simulink model "bh_1dof_and_road_sim"  (R2021b)
settings: Solver=ode15s  StartTime=0.0  StopTime=30  MaxStep=0.001  RelTol=1e-5  EnableMultiTasking=on
undefined symbols (not defined in the file or in its folder): X, Y, Z
libraries: sm_lib x22, nesl_utility x6
Description:
  | Copyright 2014 The MathWorks, Inc.
settings Model: Creator=smiller  LastModifiedBy=bhorton
settings SolverCC: AlgebraicLoopSolver=TrustRegion
settings DataIOCC: LimitDataPoints=on  SaveFormat=Array  ReturnWorkspaceOutputs=off
settings OptimizationCC: LifeSpan=inf
settings DebuggingCC: UnderspecifiedInitializationDetection=Classic  MergeDetectMultiDrivingBlocksExec=none  SolverPrmCheckMsg=warning  AllowSymbolicDim=off  StateNameClashWarn=warning  SFUnexpectedBacktrackingDiag=warning  SFNoUnconditionalDefaultTransitionDiag=warning  SFExecutionAtInitializationDiag=none  SFMachineParentedDataDiag=warning  ArithmeticOperatorsInVariantConditions=warning
settings HardwareCC: ProdBitPerPointer=32  ProdBitPerSizeT=32  ProdBitPerPtrDiffT=32  ProdLargestAtomicFloat=None  ProdIntDivRoundTo=Undefined  ProdEndianess=Unspecified  ProdWordSize=32  ProdHWDeviceType=32-bit Generic
settings ModelReferenceCC: PropagateSignalLabelsOutOfModel=off
settings SFSimCC: SimUseLocalCustomCode=off  CustomCodeUndefinedFunction=UseInterfaceOnly
settings RTWCC: RTWUseLocalCustomCode=off
settings CodeAppCC: StateflowObjectComments=on
settings GRTTargetCC: TargetLangStandard=C89/C90 (ANSI)
settings ConfigComp: CovMetricSettings=dw  CovSaveCumulativeToWorkspaceVar=on  CovSaveSingleToWorkspaceVar=on  CovExternalEMLEnable=off  CovSFcnEnable=off
settings SimscapeCC: SimscapeNormalizeSystem=off
settings ExplorerConfigSet: InternalSimMechanicsExplorerSettings="<ExplorerConfiguration><canonicalview>default</canonicalview><AnimationSetting><BasePlaybackSpeed>1.0</BasePlaybackSpeed><PlaybackSpeedFactor>0.5</PlaybackSpeedFactor></AnimationSetting><TilePanel><TileInfo><Tiles Columns=\"1\" Count=\"1\" Rows=\"1\"><Column Weight=\"1\"/><Row Weight=\"1\"/><Tile Height=\"1\" Width=\"1\" X=\"0\" Y=\"0\"/></Tiles></TileInfo><SceneInfo><SceneViewer><BGColor><R>0.60000002384185791</R><G>0.60000002384185791</G><B>0.60000002384185791</B></BGColor><Camera><DoPerspective>on</DoPerspective><Position><X>0</X><Y>0</Y><Z>3</Z></Position><Center><X>0</X><Y>0</Y><Z>0</Z></Center><Up><X>0</X><Y>1</Y><Z>0</Z></Up><ViewLimDist>1</ViewLimDist><YLim>0.466307658154998583</YLim><XLim>0.517856281102247462</XLim></Camera></SceneViewer></SceneInfo></TilePanel><MechEditorPanel><Cameras><Camera><Id>Camera1</Id><Value><Name>Camera1</Name><NativeCamera><PositionTrackingFeature>THE_MODEL.CAR_ALTERNATE_MODEL_SIMSCAPE.RF_CAM.R</PositionTrackingFeature><CenterTrackingFeature>THE_MODEL.CAR_ALTERNATE_MODEL_SIMSCAPE.Road.R</CenterTrackingFeature><UpVectorTrackingFeature>THE_MODEL.CAR_ALTERNATE_MODEL_SIMSCAPE.RF1.R</UpVectorTrackingFeature><CenterTrackingOrigin>on</CenterTrackingOrigin><UpVectorTrackingDirection>+Y</UpVectorTrackingDirection></NativeCamera></Value></Camera></Cameras><GfxPanelCameraMap><MapElement CameraMLId=\"Camera1\" GfxPanelIndex=\"0\"/></GfxPanelCameraMap><VideoCreator><PlaybackSpeedRatio>4.0</PlaybackSpeedRatio><FrameRate>30</FrameRate><VideoFormat>MPEG-4</VideoFormat><FrameSize>[400 400]</FrameSize></VideoCreator></MechEditorPanel></ExplorerConfiguration>"

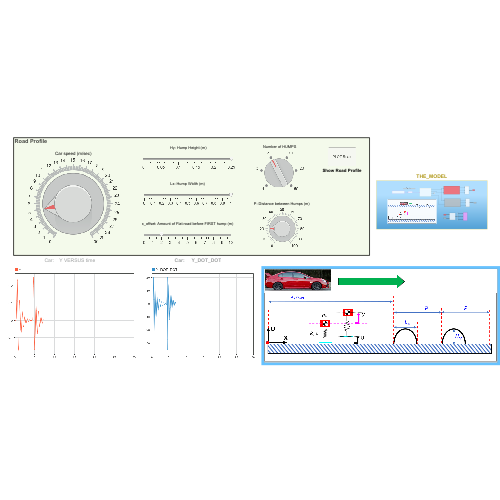
[thumbnail: Simulink's stored preview of the top-level diagram]
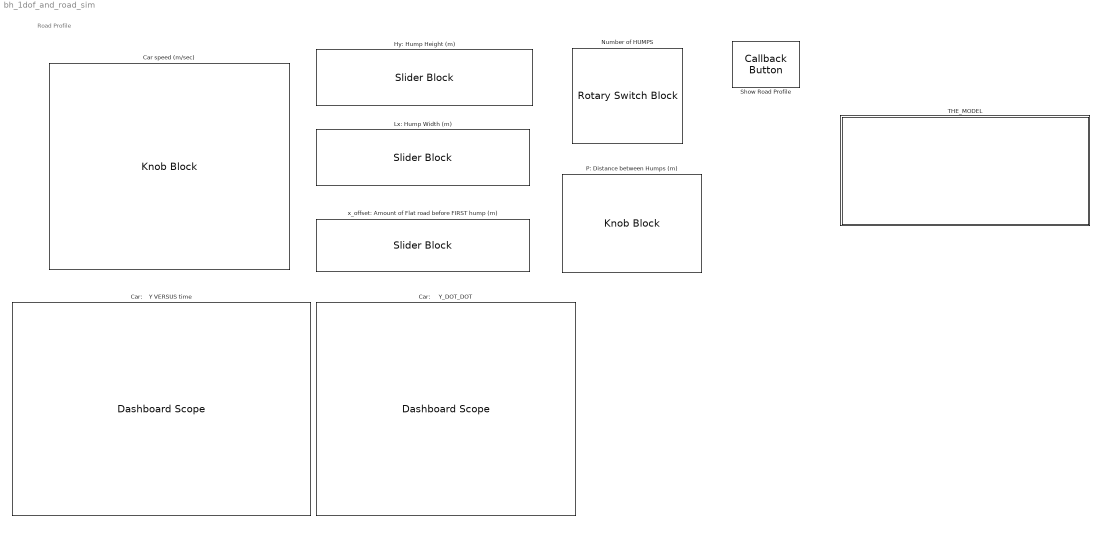
== system bh_1dof_and_road_sim ==
  note: Road Profile
  Car speed (m/sec) : KnobBlock  LabelPosition=Hide  ScaleMax=30  TickInterval=1
  Car:     Y_DOT_DOT : DashboardScope
  Car:    Y VERSUS time : DashboardScope
  Hy: Hump Height (m) : SliderBlock  LabelPosition=Hide  ScaleMax=0.25
  Lx: Hump Width (m) : SliderBlock  LabelPosition=Hide  ScaleMax=1
  Number of HUMPS : RotarySwitchBlock  LabelPosition=Hide
      settings: Values={{'1', '3', '5', '10', '20', '50'}, [1 3 5 10 20 50]}
  P: Distance between Humps (m) : KnobBlock  LabelPosition=Hide
  Show Road Profile : CallbackButton  ButtonText=PLOT Road
      settings: ClickFcn=bh_show_road_profile_from_Simulink(bdroot)
  THE_MODEL : Subsystem
  x_offset: Amount of Flat road before FIRST hump (m) : SliderBlock  LabelPosition=Hide  ScaleMax=10

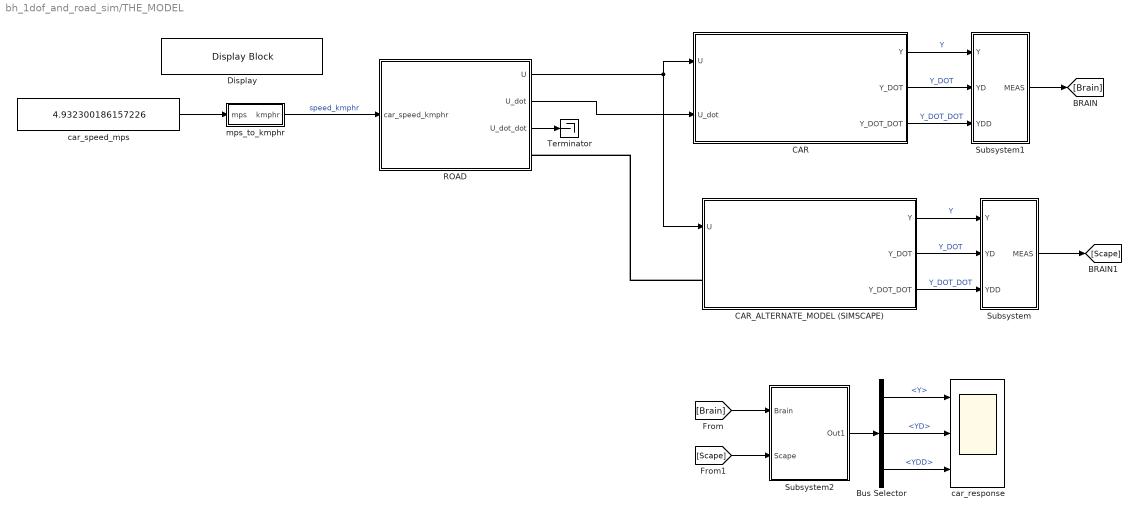
== system bh_1dof_and_road_sim/THE_MODEL ==
  Bus Selector : BusSelector  OutputSignals=Y,YD,YDD
  CAR : Subsystem  mask{m=5, c=2*10*0.6, k=500, y0=0, y_dot_0=0}
      mask prompts: m "m  (kg)"; c "c (N.s/m)"; k "k (N/m)"; y0 "y0 (m)"; y_dot_0 "y_dot_0  (m/s)"
      mask init:
      | str0 = sprintf('m  = %5.2f   (kg)', m);
      | str1 = sprintf('c  = %5.2f   (N.s/m)', c);
      | str2 = sprintf('k  = %5.2f   (N/m)', k);
      | str3 = sprintf('\n');
      | str4 = sprintf('y0 = %5.2f   (m)', y0);
      | str5 = sprintf('v0 = %5.2f   (m/s)', y_dot_0);
      | 
      | str  = char(str0,str1,str2,str3,str4,str5);
      mask DialogControl Container4 Prompt: M,C,K
      mask DialogControl Container3 Prompt: Initial Conditions
      mask Display: disp(str)
  CAR_ALTERNATE_MODEL (SIMSCAPE) : Subsystem  mask{m=5, c=2*10*0.6, k=500, y0=0, y_dot_0=0}
      mask prompts: m "m  (kg)"; c "c (N.s/m)"; k "k (N/m)"; y0 "y0 (m)"; y_dot_0 "y_dot_0  (m/s)"
      mask init: same as bh_1dof_and_road_sim/THE_MODEL/CAR
      mask DialogControl Container4 Prompt: M,C,K
      mask DialogControl Container3 Prompt: Initial Conditions
      mask Display: disp(str)
  Display : DisplayBlock  Format=short  Transparency=1
  ROAD : Subsystem  mask{m_Hy=0.25, m_Lx=1, m_P=20.15766016642253, m_x_offset=2, m_Np=5}
      mask prompts: m_Hy "Height of hump (m)"; m_Lx "Length of hump (m)"; m_P "Period of window (m)"; m_x_offset "X direction offset"; m_Np "Number of periods"
      mask init:
      | % create SYS object
      | OBJ = bh_road_hump_A_SYSO("Hy",m_Hy, "Lx",m_Lx, "P",m_P, ...
      |                           "x_offset",m_x_offset, "NUM_PERIODS",m_Np);
      |                       
      | tmp_x = linspace(0,(m_Np*m_P  +  m_x_offset), 1e4);
      | tmp_y = OBJ.get_y(tmp_x);
      | tmp_z = -2 * ones(size(tmp_x));
      | 
      | the_road_XYZ = [ tmp_x(:), tmp_y(:), tmp_z(:) ];
      mask DialogControl Control2 Prompt: Road Profile Parameters
  Subsystem : Subsystem
  Subsystem1 : Subsystem
  Subsystem2 : Subsystem
  Terminator : Terminator
  car_response : Scope  NumInputPorts=3
  car_speed_mps : Constant  Value=4.932300186157226
  mps_to_kmphr : Subsystem
  wires:
  ROAD/1(U) -> CAR/1(U), CAR_ALTERNATE_MODEL (SIMSCAPE)/1(U)
  car_speed_mps/1 -> mps_to_kmphr/1(mps)
  mps_to_kmphr/1(kmphr) -> ROAD/1(car_speed_kmphr)  "speed_kmphr"
  ROAD/2(U_dot) -> CAR/2(U_dot)
  ROAD/3(U_dot_dot) -> Terminator/1
  CAR_ALTERNATE_MODEL (SIMSCAPE)/1(Y) -> Subsystem/1(Y)  "Y"
  CAR_ALTERNATE_MODEL (SIMSCAPE)/2(Y_DOT) -> Subsystem/2(YD)  "Y_DOT"
  CAR_ALTERNATE_MODEL (SIMSCAPE)/3(Y_DOT_DOT) -> Subsystem/3(YDD)  "Y_DOT_DOT"
  CAR/1(Y) -> Subsystem1/1(Y)  "Y"
  CAR/2(Y_DOT) -> Subsystem1/2(YD)  "Y_DOT"
  CAR/3(Y_DOT_DOT) -> Subsystem1/3(YDD)  "Y_DOT_DOT"
  Subsystem1/1(MEAS) -> [Brain]
  Subsystem/1(MEAS) -> [Scape]
  [Brain] -> Subsystem2/1(Brain)
  [Scape] -> Subsystem2/2(Scape)
  Subsystem2/1(Out1) -> Bus Selector/1
  Bus Selector/1 -> car_response/1  "<Y>"
  Bus Selector/2 -> car_response/2  "<YD>"
  Bus Selector/3 -> car_response/3  "<YDD>"
  connections:
  CAR_ALTERNATE_MODEL (SIMSCAPE)/LConn1 -- ROAD/RConn1

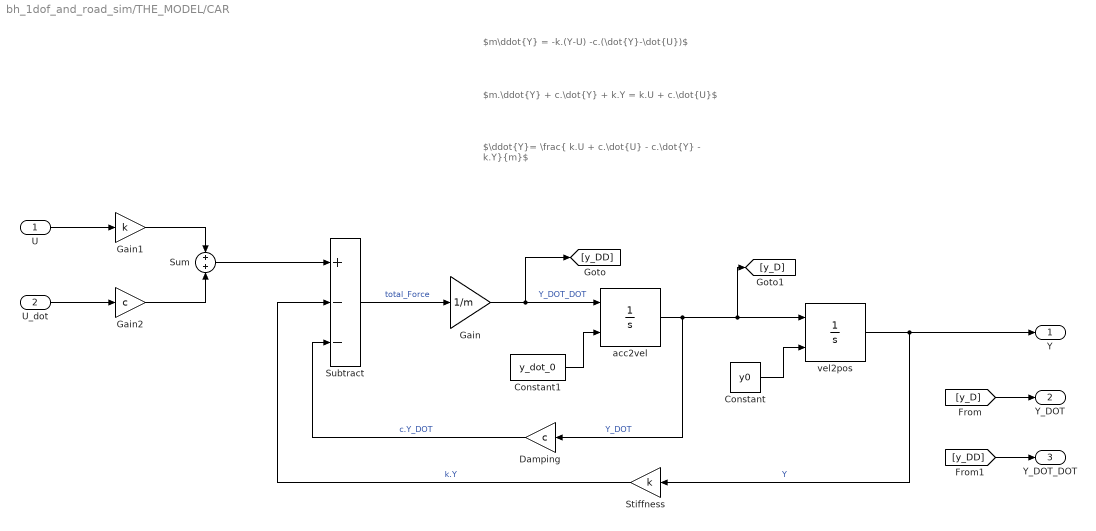
== system bh_1dof_and_road_sim/THE_MODEL/CAR ==
  note: $m.\ddot{Y} + c.\dot{Y} + k.Y = k.U + c.\dot{U}$
  note: $m\ddot{Y} = -k.(Y-U) -c.(\dot{Y}-\dot{U})$
  note: $\ddot{Y}= \frac{ k.U + c.\dot{U} - c.\dot{Y} - k.Y}{m}$
  U : Inport
  U_dot : Inport  Port=2
  Constant : Constant  Value=y0
  Constant1 : Constant  Value=y_dot_0
  Damping : Gain  Gain=c
  Gain : Gain  Gain=1/m
  Gain1 : Gain  Gain=k
  Gain2 : Gain  Gain=c
  Stiffness : Gain  Gain=k
  Subtract : Sum  Inputs=+--
  Sum : Sum  Inputs=+|+
  acc2vel : Integrator  InitialConditionSource=external
  vel2pos : Integrator  InitialConditionSource=external
  Y : Outport
  Y_DOT : Outport  Port=2
  Y_DOT_DOT : Outport  Port=3
  wires:
  Gain/1 -> [y_DD], acc2vel/1  "Y_DOT_DOT"
  Constant1/1 -> acc2vel/2
  Sum/1 -> Subtract/1
  Stiffness/1 -> Subtract/2  "k.Y"
  vel2pos/1 -> Y/1, Stiffness/1  "Y"
  Subtract/1 -> Gain/1  "total_Force"
  Constant/1 -> vel2pos/2
  acc2vel/1 -> [y_D], vel2pos/1, Damping/1  "Y_DOT"
  Damping/1 -> Subtract/3  "c.Y_DOT"
  U/1 -> Gain1/1
  U_dot/1 -> Gain2/1
  Gain1/1 -> Sum/1
  Gain2/1 -> Sum/2
  [y_D] -> Y_DOT/1
  [y_DD] -> Y_DOT_DOT/1

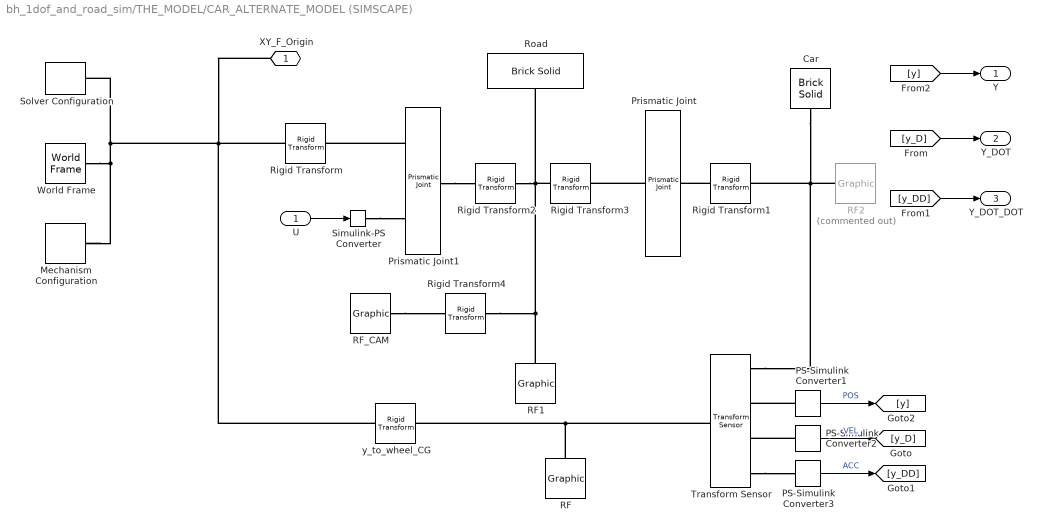
== system bh_1dof_and_road_sim/THE_MODEL/CAR_ALTERNATE_MODEL (SIMSCAPE) ==
  U : Inport
  Car : sm_lib/Body Elements/Brick Solid  GraphicAmbientColor=[0.15 0.15 0.15 1.0]  BasedOnType=Density  BrickDimensions=[1 1 1]*0.2  BrickDimensionUnits=m  CenterOfMass=[0 0 0]  CenterOfMassUnits=m  GraphicDiffuseColor=[1.0 0.2 0.2]  Density=1000  DensityUnits=kg/m^3  DoExposeReferenceFrame=on  GraphicEmissiveColor=[0.0 0.0 0.0 1.0]  ExportEntireGeometry=off  SerializedFrames=<Frames/>  MarkerShape=Sphere  MarkerSize=10  GraphicType=FromGeometry  InertiaType=PointMass  Mass=m  MassUnits=kg  MomentsOfInertia=[1 1 1]  MomentsOfInertiaUnits=kg*m^2  GraphicOpacity=1.0  ProductsOfInertia=[0 0 0]  ProductsOfInertiaUnits=kg*m^2  GraphicShininess=75  GraphicSpecularColor=[0.5 0.5 0.5 1.0]  GraphicVisPropType=SimpleVisualProperties
  Mechanism Configuration : sm_lib/Utilities/Mechanism Configuration  UniformGravity=Constant  GravityVector=[0 0 0]  GravityUnits=m/s^2  LinearizationDelta=0.001  JointModeTransitionNonlinearIterations=2
  PS-Simulink Converter1 : nesl_utility/PS-Simulink Converter  PhysicalDomain=network_engine_domain  SubClassName=ps_output  LeftPortType=input  RightPortType=output  PseudoPeriodic=off  Frequencies=[]  Unit=m  AffineConversion=off
      settings: SourceProductBaseCode=PW,SS
  PS-Simulink Converter2 : nesl_utility/PS-Simulink Converter  PhysicalDomain=network_engine_domain  SubClassName=ps_output  LeftPortType=input  RightPortType=output  PseudoPeriodic=off  Frequencies=[]  Unit=m/s  AffineConversion=off
      settings: SourceProductBaseCode=PW,SS
  PS-Simulink Converter3 : nesl_utility/PS-Simulink Converter  PhysicalDomain=network_engine_domain  SubClassName=ps_output  LeftPortType=input  RightPortType=output  PseudoPeriodic=off  Frequencies=[]  Unit=m/s^2  AffineConversion=off
      settings: SourceProductBaseCode=PW,SS
  Prismatic Joint : sm_lib/Joints/Prismatic Joint  JointMode=Normal  SenseConstraintForce=off  SenseConstraintForceX=off  SenseConstraintForceY=off  SenseConstraintForceZ=off  SenseConstraintTorque=off  SenseConstraintTorqueX=off  SenseConstraintTorqueY=off  SenseConstraintTorqueZ=off  SenseTotalForce=off  SenseTotalForceX=off  SenseTotalForceY=off  SenseTotalForceZ=off  SenseTotalTorque=off  SenseTotalTorqueX=off  SenseTotalTorqueY=off  SenseTotalTorqueZ=off  CompositeWrenchDir=FollowerOnBase  CompositeWrenchFrame=BaseFrame  EquilibriumPosition=1  EquilibriumPositionUnits=m  SpringStiffness=k  SpringStiffnessUnits=N/m  DampingCoefficient=c  DampingCoefficientUnits=N/(m/s)  TorqueActuationMode=NoTorque  MotionActuationMode=ComputedMotion  SensePosition=off  SenseVelocity=off  SenseAcceleration=off  SenseTorqueForce=off  SenseLowerLimitTorqueForce=off  SenseUpperLimitTorqueForce=off  LowerLimitSpecify=off  LowerLimitBound=-1  LowerLimitBoundUnits=m  LowerLimitStiffness=1e6  LowerLimitStiffnessUnits=N/m  LowerLimitDamping=1e3  LowerLimitDampingUnits=N/(m/s)  LowerLimitTransitionRegionWidth=1e-4  LowerLimitTransitionRegionWidthUnits=m  UpperLimitSpecify=off  UpperLimitBound=1  UpperLimitBoundUnits=m  UpperLimitStiffness=1e6  UpperLimitStiffnessUnits=N/m  UpperLimitDamping=1e3  UpperLimitDampingUnits=N/(m/s)  UpperLimitTransitionRegionWidth=1e-4  UpperLimitTransitionRegionWidthUnits=m  PositionTargetSpecify=on  PositionTargetPriority=High  PositionTargetValue=1 + y0  PositionTargetValueUnits=m  VelocityTargetSpecify=on  VelocityTargetPriority=High  VelocityTargetValue=y_dot_0  VelocityTargetValueUnits=m/s
      settings: AttributesFormatString=|
      | C = %<DampingCoefficient>
      | K = %<SpringStiffness>
      | L = %<EquilibriumPosition>
      | y0 =%<PositionTargetValue>
      | y_dot_0 = %<VelocityTargetValue>
  Prismatic Joint1 : sm_lib/Joints/Prismatic Joint  JointMode=Normal  SenseConstraintForce=off  SenseConstraintForceX=off  SenseConstraintForceY=off  SenseConstraintForceZ=off  SenseConstraintTorque=off  SenseConstraintTorqueX=off  SenseConstraintTorqueY=off  SenseConstraintTorqueZ=off  SenseTotalForce=off  SenseTotalForceX=off  SenseTotalForceY=off  SenseTotalForceZ=off  SenseTotalTorque=off  SenseTotalTorqueX=off  SenseTotalTorqueY=off  SenseTotalTorqueZ=off  CompositeWrenchDir=FollowerOnBase  CompositeWrenchFrame=BaseFrame  EquilibriumPosition=0  EquilibriumPositionUnits=m  SpringStiffness=0  SpringStiffnessUnits=N/m  DampingCoefficient=0  DampingCoefficientUnits=N/(m/s)  TorqueActuationMode=ComputedTorque  MotionActuationMode=InputMotion  SensePosition=off  SenseVelocity=off  SenseAcceleration=off  SenseTorqueForce=off  SenseLowerLimitTorqueForce=off  SenseUpperLimitTorqueForce=off  LowerLimitSpecify=off  LowerLimitBound=-1  LowerLimitBoundUnits=m  LowerLimitStiffness=1e6  LowerLimitStiffnessUnits=N/m  LowerLimitDamping=1e3  LowerLimitDampingUnits=N/(m/s)  LowerLimitTransitionRegionWidth=1e-4  LowerLimitTransitionRegionWidthUnits=m  UpperLimitSpecify=off  UpperLimitBound=1  UpperLimitBoundUnits=m  UpperLimitStiffness=1e6  UpperLimitStiffnessUnits=N/m  UpperLimitDamping=1e3  UpperLimitDampingUnits=N/(m/s)  UpperLimitTransitionRegionWidth=1e-4  UpperLimitTransitionRegionWidthUnits=m  PositionTargetSpecify=off  PositionTargetPriority=High  PositionTargetValue=0  PositionTargetValueUnits=m  VelocityTargetSpecify=off  VelocityTargetPriority=High  VelocityTargetValue=0  VelocityTargetValueUnits=m/s
  RF : sm_lib/Body Elements/Graphic  GraphicType=Marker  MarkerShape=Frame  MarkerSize=30  GraphicVisPropType=SimpleVisualProperties  GraphicDiffuseColor=[0.0 0.0 0.0]  GraphicSpecularColor=[0.5 0.5 0.5 1.0]  GraphicAmbientColor=[0.15 0.15 0.15 1.0]  GraphicEmissiveColor=[0.0 0.0 0.0 1.0]  GraphicShininess=75  GraphicOpacity=1.0
  RF1 : sm_lib/Body Elements/Graphic  GraphicType=Marker  MarkerShape=Frame  MarkerSize=30  GraphicVisPropType=SimpleVisualProperties  GraphicDiffuseColor=[0.0 0.0 0.0]  GraphicSpecularColor=[0.5 0.5 0.5 1.0]  GraphicAmbientColor=[0.15 0.15 0.15 1.0]  GraphicEmissiveColor=[0.0 0.0 0.0 1.0]  GraphicShininess=75  GraphicOpacity=1.0
  RF2 : sm_lib/Body Elements/Graphic  Commented=on  GraphicType=Marker  MarkerShape=Frame  MarkerSize=50  GraphicVisPropType=SimpleVisualProperties  GraphicDiffuseColor=[0.2 0.2 1.0]  GraphicSpecularColor=[0.5 0.5 0.5 1.0]  GraphicAmbientColor=[0.15 0.15 0.15 1.0]  GraphicEmissiveColor=[0.0 0.0 0.0 1.0]  GraphicShininess=75  GraphicOpacity=1.0
  RF_CAM : sm_lib/Body Elements/Graphic  GraphicType=Marker  MarkerShape=Frame  MarkerSize=30  GraphicVisPropType=SimpleVisualProperties  GraphicDiffuseColor=[0.0 0.0 0.0]  GraphicSpecularColor=[0.5 0.5 0.5 1.0]  GraphicAmbientColor=[0.15 0.15 0.15 1.0]  GraphicEmissiveColor=[0.0 0.0 0.0 1.0]  GraphicShininess=75  GraphicOpacity=1.0
  Rigid Transform : sm_lib/Frames and Transforms/Rigid Transform  TranslationMethod=None  TranslationStandardOffset=0  TranslationLengthUnit=m  TranslationStandardAxis=+Z  TranslationCartesianOffset=[0 0 0]  TranslationROffset=0  TranslationROffsetUnits=m  TranslationZOffset=0  TranslationZOffsetUnits=m  TranslationThetaOffset=0  TranslationThetaOffsetUnits=deg  RotationMethod=AlignedAxes  RotationAngleUnits=deg  RotationStandardAxis=+Z  RotationAngle=0.0  RotationArbitraryAxis=[0 0 1]  FollAlignAxisA=+Z  BaseAlignAxisA=+Y  FollAlignAxisB=+X  BaseAlignAxisB=+X  RotationSequenceAxes=FollowerAxes  RotationSequence=XYX  RotationSequenceAngles=[0 0 0]  RotationSequenceAnglesUnits=deg  RotationMatrix=[1 0 0; 0 1 0; 0 0 1]
  Rigid Transform1 : sm_lib/Frames and Transforms/Rigid Transform  TranslationMethod=None  TranslationStandardOffset=0  TranslationLengthUnit=m  TranslationStandardAxis=+Z  TranslationCartesianOffset=[0 0 0]  TranslationROffset=0  TranslationROffsetUnits=m  TranslationZOffset=0  TranslationZOffsetUnits=m  TranslationThetaOffset=0  TranslationThetaOffsetUnits=deg  RotationMethod=AlignedAxes  RotationAngleUnits=deg  RotationStandardAxis=+Z  RotationAngle=0.0  RotationArbitraryAxis=[0 0 1]  FollAlignAxisA=+Y  BaseAlignAxisA=+Z  FollAlignAxisB=+X  BaseAlignAxisB=+X  RotationSequenceAxes=FollowerAxes  RotationSequence=XYX  RotationSequenceAngles=[0 0 0]  RotationSequenceAnglesUnits=deg  RotationMatrix=[1 0 0; 0 1 0; 0 0 1]
  Rigid Transform2 : sm_lib/Frames and Transforms/Rigid Transform  TranslationMethod=None  TranslationStandardOffset=0  TranslationLengthUnit=m  TranslationStandardAxis=+Z  TranslationCartesianOffset=[0 0 0]  TranslationROffset=0  TranslationROffsetUnits=m  TranslationZOffset=0  TranslationZOffsetUnits=m  TranslationThetaOffset=0  TranslationThetaOffsetUnits=deg  RotationMethod=AlignedAxes  RotationAngleUnits=deg  RotationStandardAxis=+Z  RotationAngle=0.0  RotationArbitraryAxis=[0 0 1]  FollAlignAxisA=+Y  BaseAlignAxisA=+Z  FollAlignAxisB=+X  BaseAlignAxisB=+X  RotationSequenceAxes=FollowerAxes  RotationSequence=XYX  RotationSequenceAngles=[0 0 0]  RotationSequenceAnglesUnits=deg  RotationMatrix=[1 0 0; 0 1 0; 0 0 1]
  Rigid Transform3 : sm_lib/Frames and Transforms/Rigid Transform  TranslationMethod=None  TranslationStandardOffset=0  TranslationLengthUnit=m  TranslationStandardAxis=+Z  TranslationCartesianOffset=[0 0 0]  TranslationROffset=0  TranslationROffsetUnits=m  TranslationZOffset=0  TranslationZOffsetUnits=m  TranslationThetaOffset=0  TranslationThetaOffsetUnits=deg  RotationMethod=AlignedAxes  RotationAngleUnits=deg  RotationStandardAxis=+Z  RotationAngle=0.0  RotationArbitraryAxis=[0 0 1]  FollAlignAxisA=+Z  BaseAlignAxisA=+Y  FollAlignAxisB=+X  BaseAlignAxisB=+X  RotationSequenceAxes=FollowerAxes  RotationSequence=XYX  RotationSequenceAngles=[0 0 0]  RotationSequenceAnglesUnits=deg  RotationMatrix=[1 0 0; 0 1 0; 0 0 1]
  Rigid Transform4 : sm_lib/Frames and Transforms/Rigid Transform  TranslationMethod=StandardAxis  TranslationStandardOffset=3  TranslationLengthUnit=m  TranslationStandardAxis=+Z  TranslationCartesianOffset=[0 0 0]  TranslationROffset=0  TranslationROffsetUnits=m  TranslationZOffset=0  TranslationZOffsetUnits=m  TranslationThetaOffset=0  TranslationThetaOffsetUnits=deg  RotationMethod=None  RotationAngleUnits=deg  RotationStandardAxis=+Z  RotationAngle=0.0  RotationArbitraryAxis=[0 0 1]  FollAlignAxisA=+Y  BaseAlignAxisA=+Z  FollAlignAxisB=+X  BaseAlignAxisB=+X  RotationSequenceAxes=FollowerAxes  RotationSequence=XYX  RotationSequenceAngles=[0 0 0]  RotationSequenceAnglesUnits=deg  RotationMatrix=[1 0 0; 0 1 0; 0 0 1]
  Road : sm_lib/Body Elements/Brick Solid  GraphicAmbientColor=[0.15 0.15 0.15 1.0]  BasedOnType=Density  BrickDimensions=[0.2, 0.05, 0.2]  BrickDimensionUnits=m  CenterOfMass=[0 0 0]  CenterOfMassUnits=m  GraphicDiffuseColor=[0.0 1.0 1.0]  Density=1000  DensityUnits=kg/m^3  DoExposeReferenceFrame=on  GraphicEmissiveColor=[0.0 0.0 0.0 1.0]  ExportEntireGeometry=off  SerializedFrames=<Frames/>  MarkerShape=Sphere  MarkerSize=10  GraphicType=FromGeometry  InertiaType=PointMass  Mass=0.001  MassUnits=kg  MomentsOfInertia=[1 1 1]  MomentsOfInertiaUnits=kg*m^2  GraphicOpacity=1.0  ProductsOfInertia=[0 0 0]  ProductsOfInertiaUnits=kg*m^2  GraphicShininess=75  GraphicSpecularColor=[0.5 0.5 0.5 1.0]  GraphicVisPropType=SimpleVisualProperties
  Simulink-PS Converter : nesl_utility/Simulink-PS Converter  PhysicalDomain=network_engine_domain  SubClassName=ps_input  LeftPortType=input  RightPortType=output  PseudoPeriodic=off  Frequencies=[]  NoiseDistribution=none  NoiseParameters=[]  Unit=m  AffineConversion=off  FilteringAndDerivatives=filter  SimscapeFilterOrder=2  InputFilterTimeConstant=0.0005  UdotUserProvided=0
      settings: SourceProductBaseCode=PW,SS
  Solver Configuration : nesl_utility/Solver Configuration  PhysicalDomain=network_engine_domain  SubClassName=solver  LeftPortType=input  RightPortType=generic  Tones=[]  Harmonics=[]  SimulateNoise=off  Profile=off  UseLocalSampling=off  EnableSwitchedLinearOptims=on  FrequencyDomain=off  UseCCode=off  RelTol=0.001  AbsTol=1e-06  MinStep=1e-09  ToWorkspace=off  RevertToSquareIcSolve=off  NumHomotopyIterations=100  PhasorMode=off  PhasorModeNumHarmonics=1  DoDC=off  ResidualTolerance=1e-09  UseLocalSolver=off  LocalSolverChoice=NE_BACKWARD_EULER_ADVANCER  LocalSolverSampleTime=0.001  DoFixedCost=off  MaxNonlinIter=3  MaxModeIter=2  ComputeImpulses=off  ImpulseIterations=2  LinearAlgebra=Sparse  EquationFormulation=NE_TIME_EF  DelaysMemoryBudget=1024  AutomaticFiltering=on  FilteringTimeConstant=0.001  PartitionStorageMethod=AS_NEEDED  PartitionMemoryBudget=1024  PartitionMethod=FAST
      settings: SourceProductBaseCode=PW,SS
  Transform Sensor : sm_lib/Frames and Transforms/Transform Sensor  MeasurementFrame=World  SenseAngle=off  SenseAxis=off  SenseAngle1=off  SenseAngle2=off  SenseAngle3=off  SenseQ=off  SenseR=off  SenseOmegaX=off  SenseOmegaY=off  SenseOmegaZ=off  SenseOmega1=off  SenseOmega2=off  SenseOmega3=off  SenseQDot=off  SenseRDot=off  SenseAlphaX=off  SenseAlphaY=off  SenseAlphaZ=off  SenseAlpha1=off  SenseAlpha2=off  SenseAlpha3=off  SenseQDDot=off  SenseRDDot=off  SenseX=off  SenseY=on  SenseZ=off  SenseRad=off  SenseAzim=off  SenseDist=off  SenseInc=off  SenseXDot=off  SenseYDot=on  SenseZDot=off  SenseRadDot=off  SenseAzimDot=off  SenseDistDot=off  SenseIncDot=off  SenseXDDot=off  SenseYDDot=on  SenseZDDot=off  SenseRadDDot=off  SenseAzimDDot=off  SenseDistDDot=off  SenseIncDDot=off
  World Frame : sm_lib/Frames and Transforms/World Frame
  y_to_wheel_CG : sm_lib/Frames and Transforms/Rigid Transform  TranslationMethod=StandardAxis  TranslationStandardOffset=1  TranslationLengthUnit=m  TranslationStandardAxis=+Y  TranslationCartesianOffset="[-0.5,  1,  0]"  TranslationROffset=0  TranslationROffsetUnits=m  TranslationZOffset=0  TranslationZOffsetUnits=m  TranslationThetaOffset=0  TranslationThetaOffsetUnits=deg  RotationMethod=None  RotationAngleUnits=deg  RotationStandardAxis=+Z  RotationAngle=0.0  RotationArbitraryAxis=[0 0 1]  FollAlignAxisA=+Z  BaseAlignAxisA=+Y  FollAlignAxisB=+X  BaseAlignAxisB=+X  RotationSequenceAxes=FollowerAxes  RotationSequence=XYX  RotationSequenceAngles=[0 0 0]  RotationSequenceAnglesUnits=deg  RotationMatrix=[1 0 0; 0 1 0; 0 0 1]
      settings: AttributesFormatString=|
      | Axis = %<TranslationStandardAxis>
      | offset = %<TranslationStandardOffset>
  XY_F_Origin : PMIOPort  Side=Left
  Y : Outport
  Y_DOT : Outport  Port=2
  Y_DOT_DOT : Outport  Port=3
  wires:
  [y_D] -> Y_DOT/1
  [y_DD] -> Y_DOT_DOT/1
  PS-Simulink Converter2/1 -> [y_D]  "VEL"
  PS-Simulink Converter3/1 -> [y_DD]  "ACC"
  PS-Simulink Converter1/1 -> [y]  "POS"
  [y] -> Y/1
  U/1 -> Simulink-PS Converter/1
  connections:
  Prismatic Joint1/LConn1 -- Rigid Transform/RConn1
  Road/RConn1 -- Rigid Transform4/LConn1 -- RF1/RConn1 -- Rigid Transform2/RConn1 -- Rigid Transform3/LConn1
  Rigid Transform1/LConn1 -- Prismatic Joint/RConn1
  Car/RConn1 -- RF2/RConn1 -- Transform Sensor/RConn1 -- Rigid Transform1/RConn1
  y_to_wheel_CG/RConn1 -- Transform Sensor/LConn1 -- RF/RConn1
  PS-Simulink Converter1/LConn1 -- Transform Sensor/RConn2
  PS-Simulink Converter2/LConn1 -- Transform Sensor/RConn3
  Transform Sensor/RConn4 -- PS-Simulink Converter3/LConn1
  Simulink-PS Converter/RConn1 -- Prismatic Joint1/LConn2
  Prismatic Joint1/RConn1 -- Rigid Transform2/LConn1
  Prismatic Joint/LConn1 -- Rigid Transform3/RConn1
  Mechanism Configuration/RConn1 -- XY_F_Origin/RConn1 -- y_to_wheel_CG/LConn1 -- Rigid Transform/LConn1 -- Solver Configuration/RConn1 -- World Frame/RConn1
  RF_CAM/RConn1 -- Rigid Transform4/RConn1

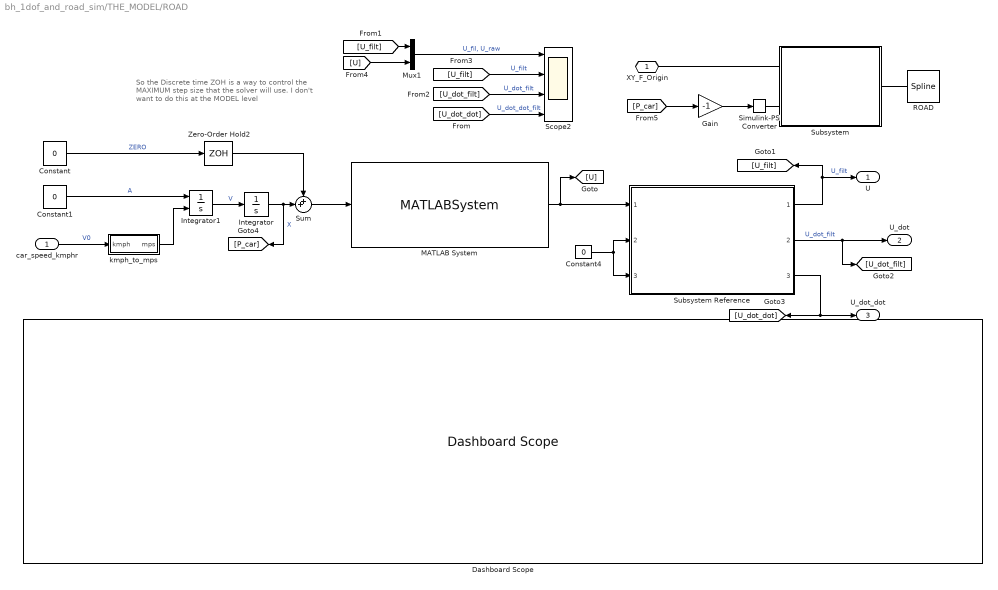
== system bh_1dof_and_road_sim/THE_MODEL/ROAD ==
  note: So the Discrete time ZOH is a way to control
      | the MAXIMUM step size that the solver will use.
      |
      | I don't want to do this at the MODEL level
  car_speed_kmphr : Inport
  Constant : Constant  Value=0
  Constant1 : Constant  Value=0
  Constant4 : Constant  Value=0
  Dashboard Scope : DashboardScope
  Gain : Gain  Gain=-1
  Integrator : Integrator
  Integrator1 : Integrator  InitialConditionSource=external
  MATLAB System : MATLABSystem  System=bh_road_hump_A_SYSO  Hy=m_Hy  Lx=m_Lx  P=m_P  x_offset=m_x_offset  NUM_PERIODS=m_Np  SimulateUsing=Interpreted execution
      mask Type: bh_road_hump_A_SYSO
      mask Display:
      | disp('bh_road_hump_A_SYSO');
      | port_label('input',1,'X_car');
      | port_label('output',1,'Y_road');
  Mux1 : Mux  Inputs=2
  ROAD : sm_lib/Curves and Surfaces/Spline  GraphicAmbientColor=[0.15 0.15 0.15 1.0]  GraphicDiffuseColor=[0.2 1.0 0.2]  DataPoints=the_road_XYZ  DataPointsUnits=m  GraphicEmissiveColor=[0.0 0.0 0.0 1.0]  EndConditionType=Natural  MarkerShape=Sphere  MarkerSize=10  GraphicType=FromGeometry  GraphicOpacity=1.0  GraphicShininess=75  GraphicSpecularColor=[0.5 0.5 0.5 1.0]  GraphicVisPropType=SimpleVisualProperties
  Scope2 : Scope  NumInputPorts=4
  Simulink-PS Converter : nesl_utility/Simulink-PS Converter  PhysicalDomain=network_engine_domain  SubClassName=ps_input  LeftPortType=input  RightPortType=output  PseudoPeriodic=off  Frequencies=[]  NoiseDistribution=none  NoiseParameters=[]  Unit=m  AffineConversion=off  FilteringAndDerivatives=filter  SimscapeFilterOrder=2  InputFilterTimeConstant=0.001  UdotUserProvided=0
      settings: SourceProductBaseCode=PW,SS
  Subsystem : Subsystem
  Subsystem Reference : Subsystem  ReferencedSubsystem=bh_COMPONENT_deriv_est  wn=2*pi*1000  p=1
  Sum : Sum  Inputs=++|
  Zero-Order Hold2 : ZeroOrderHold  SampleTime=1/1000
      settings: AttributesFormatString=dT =%<SampleTime>
  kmph_to_mps : Subsystem
  XY_F_Origin : PMIOPort  Side=Right
  U : Outport
  U_dot : Outport  Port=2
  U_dot_dot : Outport  Port=3
  wires:
  Integrator/1 -> [P_car], Sum/2  "X"
  Mux1/1 -> Scope2/1  "U_fil, U_raw"
  Sum/1 -> MATLAB System/1
  Constant1/1 -> Integrator1/1  "A"
  Constant/1 -> Zero-Order Hold2/1  "ZERO"
  MATLAB System/1 -> [U], Subsystem Reference/1
  Integrator1/1 -> Integrator/1  "V"
  kmph_to_mps/1(mps) -> Integrator1/2
  car_speed_kmphr/1 -> kmph_to_mps/1(kmph)  "V0"
  Zero-Order Hold2/1 -> Sum/1
  Constant4/1 -> Subsystem Reference/3, Subsystem Reference/2
  Subsystem Reference/2 -> U_dot/1, [U_dot_filt]  "U_dot_filt"
  Subsystem Reference/1 -> U/1, [U_filt]  "U_filt"
  [U] -> Mux1/2
  [U_filt] -> Mux1/1
  [U_filt] -> Scope2/2  "U_filt"
  [U_dot_filt] -> Scope2/3  "U_dot_filt"
  Subsystem Reference/3 -> U_dot_dot/1, [U_dot_dot]
  [U_dot_dot] -> Scope2/4  "U_dot_dot_filt"
  [P_car] -> Gain/1
  Gain/1 -> Simulink-PS Converter/1
  connections:
  Subsystem/LConn1 -- XY_F_Origin/RConn1
  Simulink-PS Converter/RConn1 -- Subsystem/LConn2
  ROAD/LConn1 -- Subsystem/RConn1

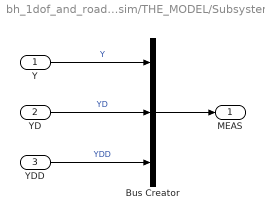
== system bh_1dof_and_road_sim/THE_MODEL/Subsystem ==
  Y : Inport
  YD : Inport  Port=2
  YDD : Inport  Port=3
  Bus Creator : BusCreator  Inputs=3
  MEAS : Outport
  wires:
  YD/1 -> Bus Creator/2  "YD"
  YDD/1 -> Bus Creator/3  "YDD"
  Y/1 -> Bus Creator/1  "Y"
  Bus Creator/1 -> MEAS/1

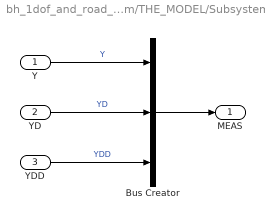
== system bh_1dof_and_road_sim/THE_MODEL/Subsystem1 ==
  Y : Inport
  YD : Inport  Port=2
  YDD : Inport  Port=3
  Bus Creator : BusCreator  Inputs=3
  MEAS : Outport
  wires:
  YD/1 -> Bus Creator/2  "YD"
  YDD/1 -> Bus Creator/3  "YDD"
  Y/1 -> Bus Creator/1  "Y"
  Bus Creator/1 -> MEAS/1

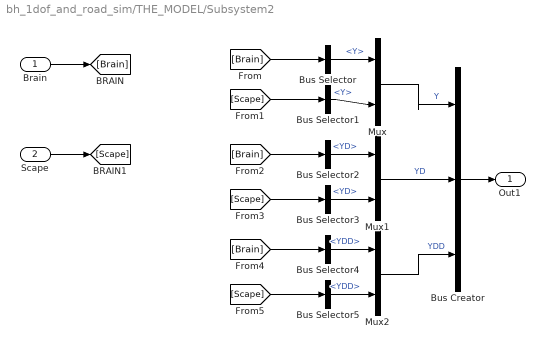
== system bh_1dof_and_road_sim/THE_MODEL/Subsystem2 ==
  Brain : Inport
  Scape : Inport  Port=2
  Bus Creator : BusCreator  Inputs=3
  Bus Selector : BusSelector  OutputSignals=Y
  Bus Selector1 : BusSelector  OutputSignals=Y
  Bus Selector2 : BusSelector  OutputSignals=YD
  Bus Selector3 : BusSelector  OutputSignals=YD
  Bus Selector4 : BusSelector  OutputSignals=YDD
  Bus Selector5 : BusSelector  OutputSignals=YDD
  Mux : Mux  Inputs=2
  Mux1 : Mux  Inputs=2
  Mux2 : Mux  Inputs=2
  Out1 : Outport
  wires:
  Scape/1 -> [Scape]
  Brain/1 -> [Brain]
  [Brain] -> Bus Selector/1
  [Scape] -> Bus Selector1/1
  Bus Selector/1 -> Mux/1  "<Y>"
  Bus Selector1/1 -> Mux/2  "<Y>"
  Bus Selector2/1 -> Mux1/1  "<YD>"
  [Brain] -> Bus Selector2/1
  [Scape] -> Bus Selector3/1
  Bus Selector3/1 -> Mux1/2  "<YD>"
  Bus Selector4/1 -> Mux2/1  "<YDD>"
  [Brain] -> Bus Selector4/1
  [Scape] -> Bus Selector5/1
  Bus Selector5/1 -> Mux2/2  "<YDD>"
  Mux1/1 -> Bus Creator/2  "YD"
  Mux/1 -> Bus Creator/1  "Y"
  Mux2/1 -> Bus Creator/3  "YDD"
  Bus Creator/1 -> Out1/1

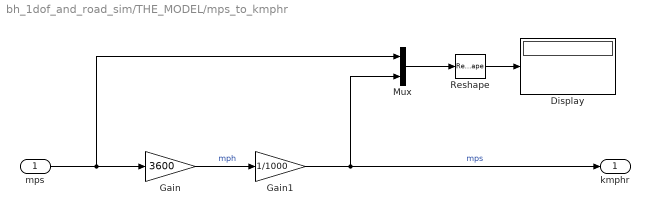
== system bh_1dof_and_road_sim/THE_MODEL/mps_to_kmphr ==
  mps : Inport
  Display : Display
  Gain : Gain  Gain=3600
  Gain1 : Gain  Gain=1/1000
  Mux : Mux  Inputs=2
  Reshape : Reshape  OutputDimensionality=Column vector (2-D)
  kmphr : Outport
  wires:
  mps/1 -> Mux/1, Gain/1
  Gain/1 -> Gain1/1  "mph"
  Gain1/1 -> Mux/2, kmphr/1  "mps"
  Reshape/1 -> Display/1
  Mux/1 -> Reshape/1

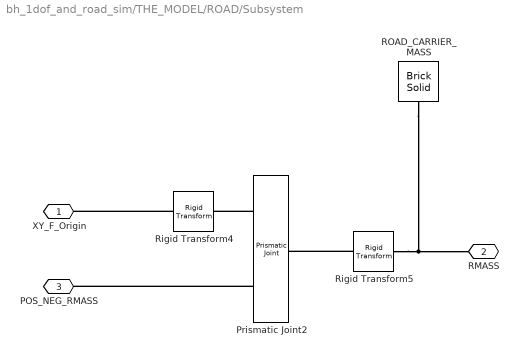
== system bh_1dof_and_road_sim/THE_MODEL/ROAD/Subsystem ==
  Prismatic Joint2 : sm_lib/Joints/Prismatic Joint  JointMode=Normal  SenseConstraintForce=off  SenseConstraintForceX=off  SenseConstraintForceY=off  SenseConstraintForceZ=off  SenseConstraintTorque=off  SenseConstraintTorqueX=off  SenseConstraintTorqueY=off  SenseConstraintTorqueZ=off  SenseTotalForce=off  SenseTotalForceX=off  SenseTotalForceY=off  SenseTotalForceZ=off  SenseTotalTorque=off  SenseTotalTorqueX=off  SenseTotalTorqueY=off  SenseTotalTorqueZ=off  CompositeWrenchDir=FollowerOnBase  CompositeWrenchFrame=BaseFrame  EquilibriumPosition=0  EquilibriumPositionUnits=m  SpringStiffness=0  SpringStiffnessUnits=N/m  DampingCoefficient=0  DampingCoefficientUnits=N/(m/s)  TorqueActuationMode=ComputedTorque  MotionActuationMode=InputMotion  SensePosition=off  SenseVelocity=off  SenseAcceleration=off  SenseTorqueForce=off  SenseLowerLimitTorqueForce=off  SenseUpperLimitTorqueForce=off  LowerLimitSpecify=off  LowerLimitBound=-1  LowerLimitBoundUnits=m  LowerLimitStiffness=1e6  LowerLimitStiffnessUnits=N/m  LowerLimitDamping=1e3  LowerLimitDampingUnits=N/(m/s)  LowerLimitTransitionRegionWidth=1e-4  LowerLimitTransitionRegionWidthUnits=m  UpperLimitSpecify=off  UpperLimitBound=1  UpperLimitBoundUnits=m  UpperLimitStiffness=1e6  UpperLimitStiffnessUnits=N/m  UpperLimitDamping=1e3  UpperLimitDampingUnits=N/(m/s)  UpperLimitTransitionRegionWidth=1e-4  UpperLimitTransitionRegionWidthUnits=m  PositionTargetSpecify=off  PositionTargetPriority=High  PositionTargetValue=0  PositionTargetValueUnits=m  VelocityTargetSpecify=off  VelocityTargetPriority=High  VelocityTargetValue=0  VelocityTargetValueUnits=m/s
  ROAD_CARRIER_MASS : sm_lib/Body Elements/Brick Solid  GraphicAmbientColor=[0.15 0.15 0.15 1.0]  BasedOnType=Density  BrickDimensions=[1, 1, 1]/100  BrickDimensionUnits=m  CenterOfMass=[0 0 0]  CenterOfMassUnits=m  GraphicDiffuseColor=[0.0 0.8 0.2]  Density=1000  DensityUnits=kg/m^3  DoExposeReferenceFrame=on  GraphicEmissiveColor=[0.0 0.0 0.0 1.0]  ExportEntireGeometry=off  SerializedFrames=<Frames/>  MarkerShape=Sphere  MarkerSize=10  GraphicType=FromGeometry  InertiaType=PointMass  Mass=1  MassUnits=kg  MomentsOfInertia=[1 1 1]  MomentsOfInertiaUnits=kg*m^2  GraphicOpacity=1.0  ProductsOfInertia=[0 0 0]  ProductsOfInertiaUnits=kg*m^2  GraphicShininess=75  GraphicSpecularColor=[0.5 0.5 0.5 1.0]  GraphicVisPropType=SimpleVisualProperties
  Rigid Transform4 : sm_lib/Frames and Transforms/Rigid Transform  TranslationMethod=None  TranslationStandardOffset=0  TranslationLengthUnit=m  TranslationStandardAxis=+Z  TranslationCartesianOffset=[0 0 0]  TranslationROffset=0  TranslationROffsetUnits=m  TranslationZOffset=0  TranslationZOffsetUnits=m  TranslationThetaOffset=0  TranslationThetaOffsetUnits=deg  RotationMethod=AlignedAxes  RotationAngleUnits=deg  RotationStandardAxis=+Z  RotationAngle=0.0  RotationArbitraryAxis=[0 0 1]  FollAlignAxisA=+Z  BaseAlignAxisA=+X  FollAlignAxisB=+Y  BaseAlignAxisB=+Y  RotationSequenceAxes=FollowerAxes  RotationSequence=XYX  RotationSequenceAngles=[0 0 0]  RotationSequenceAnglesUnits=deg  RotationMatrix=[1 0 0; 0 1 0; 0 0 1]
  Rigid Transform5 : sm_lib/Frames and Transforms/Rigid Transform  TranslationMethod=None  TranslationStandardOffset=0  TranslationLengthUnit=m  TranslationStandardAxis=+Z  TranslationCartesianOffset=[0 0 0]  TranslationROffset=0  TranslationROffsetUnits=m  TranslationZOffset=0  TranslationZOffsetUnits=m  TranslationThetaOffset=0  TranslationThetaOffsetUnits=deg  RotationMethod=AlignedAxes  RotationAngleUnits=deg  RotationStandardAxis=+Z  RotationAngle=0.0  RotationArbitraryAxis=[0 0 1]  FollAlignAxisA=+X  BaseAlignAxisA=+Z  FollAlignAxisB=+Y  BaseAlignAxisB=+Y  RotationSequenceAxes=FollowerAxes  RotationSequence=XYX  RotationSequenceAngles=[0 0 0]  RotationSequenceAnglesUnits=deg  RotationMatrix=[1 0 0; 0 1 0; 0 0 1]
  XY_F_Origin : PMIOPort  Side=Left
  RMASS : PMIOPort  Port=2  Side=Right
  POS_NEG_RMASS : PMIOPort  Port=3  Side=Left
  connections:
  Prismatic Joint2/LConn1 -- Rigid Transform4/RConn1
  Rigid Transform5/LConn1 -- Prismatic Joint2/RConn1
  Prismatic Joint2/LConn2 -- POS_NEG_RMASS/RConn1
  Rigid Transform4/LConn1 -- XY_F_Origin/RConn1
  Rigid Transform5/RConn1 -- ROAD_CARRIER_MASS/RConn1 -- RMASS/RConn1

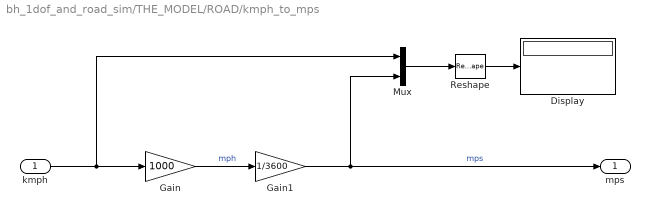
== system bh_1dof_and_road_sim/THE_MODEL/ROAD/kmph_to_mps ==
  kmph : Inport
  Display : Display
  Gain : Gain  Gain=1000
  Gain1 : Gain  Gain=1/3600
  Mux : Mux  Inputs=2
  Reshape : Reshape  OutputDimensionality=Column vector (2-D)
  mps : Outport
  wires:
  kmph/1 -> Mux/1, Gain/1
  Gain/1 -> Gain1/1  "mph"
  Gain1/1 -> Mux/2, mps/1  "mps"
  Reshape/1 -> Display/1
  Mux/1 -> Reshape/1
